simulink model "Continuous3"  (R2020a)
settings: Solver=VariableStepAuto  StartTime=0.0  StopTime=2  FixedStep=0.1  RelTol=1e-3  EnableMultiTasking=on
settings Model: Creator=BEAR  LastModifiedBy=bzhan
settings SolverCC: AutoInsertRateTranBlk=on
settings DataIOCC: LimitDataPoints=on  ReturnWorkspaceOutputs=off
settings OptimizationCC: LifeSpan=inf
settings DebuggingCC: AllowSymbolicDim=off  SFUnexpectedBacktrackingDiag=warning  SFNoUnconditionalDefaultTransitionDiag=warning  SFExecutionAtInitializationDiag=none  ArithmeticOperatorsInVariantConditions=warning
settings SFSimCC: SimUseLocalCustomCode=off  CustomCodeUndefinedFunction=UseInterfaceOnly
settings RTWCC: RTWUseLocalCustomCode=off
settings CodeAppCC: StateflowObjectComments=on
settings GRTTargetCC: TargetLangStandard=C89/C90 (ANSI)
settings ConfigComp: CovMetricSettings=dw  CovHtmlReporting=on  CovSaveCumulativeToWorkspaceVar=on  CovSaveSingleToWorkspaceVar=on  CovShowResultsExplorer=off  CovExternalEMLEnable=off  CovSFcnEnable=off

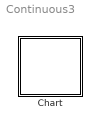
== system Continuous3 ==
  Chart : Stateflow chart  TreatAsAtomicUnit=on

== stateflow chart Continuous3/Chart ==
  settings: updateMethod=CONTINUOUS
  state A
    en: f("enA")
    du: x_dot=1; y_dot=x;
    ex: f("exA")
  state B
    en: f("enB"); x=0;
    du: x_dot=1;
    state B1
      en: f("enB1")
    (default) -> B1
  (default) -> A : {x=0;y=0;}
  A -> B1 : [y >= 1]{f("conAB1")}/{f("tranAB1")}
  B -> B : [x>=1]
  data: s function_input; y local double; x local double
  data y settings: updateMethod=SF_CONTINUOUS_TIME_DATA
  data x settings: updateMethod=SF_CONTINUOUS_TIME_DATA
  function f(s):
    | function f(s)
    |     fprintf(s+' %.3f %.3f\n', x, y);
